simulink model "QuinReader_HW"  (R2023b)
settings: Solver=FixedStepDiscrete  StartTime=0.0  StopTime=5e5*SAMPLE_TIME  RelTol=1e-3
InitFcn:
  | Initialize;
values from neighbouring files (symbols this model uses):
  ALIGN_SIG_LEN = 5000    [Initialize.m]
  BLF = 40e3    (= 40000)    [Initialize.m]
  LPBACK_DECI = designMultirateFIR(1, 2, 0.25, 60,"SystemObject", true)    [Initialize.m]
  NCO = gen_nco_config(SAMPLE_RATE, OperateFreq - CenterFreq)    [Initialize.m]
  SAMPLE_RATE = 122.88e6    (= 122880000)    [Initialize.m]
  SAMPLE_TIME = 1 / SAMPLE_RATE    (= 8.13802083333e-09)    [Initialize.m]
  TX_INTER = designMultirateFIR(2, 1, 0.25, 60,"SystemObject", true)    [Initialize.m]
undefined symbols (not defined in the file or in its folder): ReaderReceive
libraries: hdlsllib x16, simulink x5, dsphdlsigops2 x5, dsphdlfiltering2 x2
CloseFcn:
  | clear rfid rn16 epc rn16_start epc_start
settings Model: DataTypeOverride=Off  Creator=NaXin  LastModifiedBy=NaXin
settings SolverCC: AlgebraicLoopSolver=TrustRegion
settings DataIOCC: LimitDataPoints=on  SaveOutput=off  SaveTime=off
settings OptimizationCC: BlockReduction=off  ConditionallyExecuteInputs=off  DefaultParameterBehavior=Inlined  InheritOutputTypeSmallerThanSingle=on  ReuseModelBlockBuffer=off  LifeSpan=inf
settings DebuggingCC: AlgebraicLoopMsg=error  SingleTaskRateTransMsg=error  UnconnectedInputMsg=warning  UnconnectedOutputMsg=warning  UnconnectedLineMsg=warning  AllowSymbolicDim=off  StrictBusMsg=ErrorOnBusTreatedAsVector  SFUnexpectedBacktrackingDiag=warning  SFNoUnconditionalDefaultTransitionDiag=warning  SFExecutionAtInitializationDiag=none  ArithmeticOperatorsInVariantConditions=warning
settings HardwareCC: ProdBitPerPointer=32  ProdBitPerSizeT=32  ProdBitPerPtrDiffT=32  ProdLargestAtomicFloat=None  ProdIntDivRoundTo=Undefined  ProdEndianess=Unspecified  ProdWordSize=32  ProdHWDeviceType=ASIC/FPGA->ASIC/FPGA  ProdEqTarget=off
settings ModelReferenceCC: EnableRefExpFcnMdlSchedulingChecks=on
settings SFSimCC: SimUseLocalCustomCode=off  CustomCodeUndefinedFunction=UseInterfaceOnly
settings RTWCC: RTWUseLocalCustomCode=off
settings CodeAppCC: StateflowObjectComments=on
settings GRTTargetCC: TargetLangStandard=C89/C90 (ANSI)
settings ConfigComp: CovScope=ReferencedModels  CovMetricSettings=dw  CovSaveCumulativeToWorkspaceVar=on  CovSaveSingleToWorkspaceVar=on  CovExternalEMLEnable=off  CovSFcnEnable=off

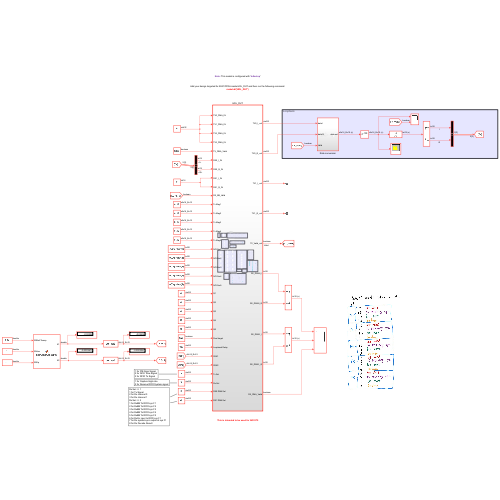
[thumbnail: Simulink's stored preview of the top-level diagram]
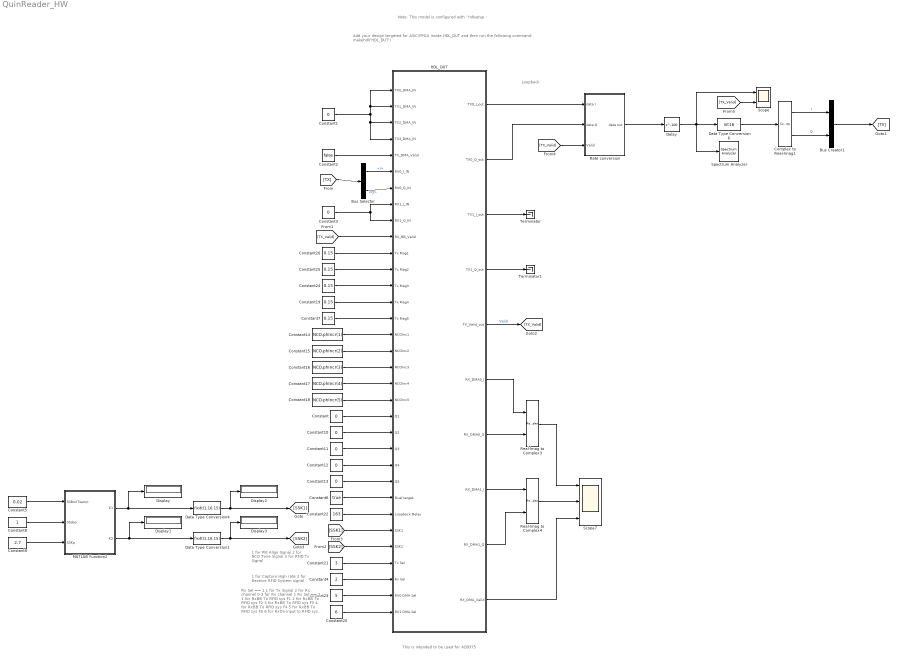
== system QuinReader_HW ==
  note: Note: This model is configured with ' hdlsetup '
  note: Add your design targeted for ASIC/FPGA inside HDL_DUT and then run the following command:
      | makehdl('HDL_DUT')
  note: Rx Sel == 1
      | 1 for Tx Signal
      | 2 for Rx channel 0
      | 3 for Rx channel 1
      | Rx Sel == 2
      | 1 for RxBB To RFID sys F1
      | 2 for RxBB To RFID sys F2
      | 3 for RxBB To RFID sys F3
      | 4 for RxBB To RFID sys F4
      | 5 for RxBB To RFID sys F5
      | 6 for RxOn input to RFID sys F1
      | 7 for Rx symbol sync output at sys F1
      | 8 for Rx Decode Result
  note: 1 for PIE Align Signal
      | 2 for NCO Tone Signal
      | 3 for RFID Tx Signal
  note: Loopback
  note: This is intended to be used for AD9375
  note: 1 for Capture High rate
      | 2 for Receive RFID System signal
  Bus Creator1 : BusCreator  Inputs=2
  Bus Selector : BusSelector  OutputSignals=I,Q
  Complex to Real-Imag1 : ComplexToRealImag
  Constant{,1,10..13} (6 alike) : Constant  Value=0  OutDataTypeStr=uint32  SampleTime=SAMPLE_TIME
  Constant14 : Constant  Value=NCO.phIncr(1)  OutDataTypeStr=int32  SampleTime=SAMPLE_TIME
  Constant15 : Constant  Value=NCO.phIncr(2)  OutDataTypeStr=int32  SampleTime=SAMPLE_TIME
  Constant16 : Constant  Value=NCO.phIncr(3)  OutDataTypeStr=int32  SampleTime=SAMPLE_TIME
  Constant17 : Constant  Value=NCO.phIncr(4)  OutDataTypeStr=int32  SampleTime=SAMPLE_TIME
  Constant18 : Constant  Value=NCO.phIncr(5)  OutDataTypeStr=int32  SampleTime=SAMPLE_TIME
  Constant{7,19,24..26} (5 alike) : Constant  Value=0.15  OutDataTypeStr=fixdt(1,16,15)  SampleTime=SAMPLE_TIME
  Constant2 : Constant  Value=false  OutDataTypeStr=boolean  SampleTime=SAMPLE_TIME
  Constant20 : Constant  Value=6  OutDataTypeStr=uint32  SampleTime=SAMPLE_TIME
  Constant21 : Constant  Value=3  OutDataTypeStr=uint32  SampleTime=SAMPLE_TIME
  Constant22 : Constant  Value=163  OutDataTypeStr=uint32  SampleTime=SAMPLE_TIME
  Constant23 : Constant  Value=5  OutDataTypeStr=uint32  SampleTime=SAMPLE_TIME
  Constant3 : Constant  Value=0  OutDataTypeStr=int16  SampleTime=SAMPLE_TIME
  Constant4 : Constant  Value=2  OutDataTypeStr=uint32  SampleTime=SAMPLE_TIME
  Constant5 : Constant  Value=0.02  SampleTime=SAMPLE_TIME
  Constant6 : Constant  Value=true  OutDataTypeStr=boolean  SampleTime=SAMPLE_TIME
  Constant8 : Constant  SampleTime=SAMPLE_TIME
  Constant9 : Constant  Value=2.7  SampleTime=SAMPLE_TIME
  Data Type Conversion1 : DataTypeConversion  OutDataTypeStr=fixdt(1,16,15)  SaturateOnIntegerOverflow=off  RndMeth=Floor
  Data Type Conversion4 : DataTypeConversion  OutDataTypeStr=fixdt(1,16,15)  SaturateOnIntegerOverflow=off  RndMeth=Floor
  Data Type Conversion6 : DataTypeConversion  OutDataTypeStr=int16  ConvertRealWorld=Stored Integer (SI)  SaturateOnIntegerOverflow=off  RndMeth=Floor
  Delay : Delay  DelayLength=100
  Display{,1..3} (4 alike) : Display
  HDL_DUT : Subsystem  TreatAsAtomicUnit=on
  MATLAB Function2 : MATLAB Function  TreatAsAtomicUnit=on
  Rate conversion : Subsystem
  Real-Imag to Complex3 : RealImagToComplex
  Real-Imag to Complex4 : RealImagToComplex
  Scope : Scope  NumInputPorts=2
  Scope7 : Scope  NumInputPorts=3
  Spectrum Analyzer : SpectrumAnalyzer  WindowPosition=[605.000000,336.000000,800.000000,500.000000,]  ScopeFrameLocation=window  Span=122880000  StartFrequency=-61440000  StopFrequency=61440000  YLimits=[-115.87985262,25.05534256]
      settings: OpenAtSimulationStart=off
  Terminator : Terminator
  Terminator1 : Terminator
  wires:
  Constant2/1 -> HDL_DUT/5(TX_DMA_Valid)
  Constant1/1 -> HDL_DUT/3(TX2_DMA_IN), HDL_DUT/4(TX3_DMA_IN), HDL_DUT/2(TX1_DMA_IN), HDL_DUT/1(TX0_DMA_IN)
  Bus Selector/2 -> HDL_DUT/7(RX0_Q_IN)  "<Q>"
  [TX] -> Bus Selector/1
  Bus Selector/1 -> HDL_DUT/6(RX0_I_IN)  "<I>"
  Constant3/1 -> HDL_DUT/9(RX1_Q_IN), HDL_DUT/8(RX1_I_IN)
  Constant7/1 -> HDL_DUT/15(Tx Mag5)
  Constant/1 -> HDL_DUT/21(Q1)
  Constant20/1 -> HDL_DUT/33(RX1 DMA Sel)
  Constant23/1 -> HDL_DUT/32(RX0 DMA Sel)
  Constant21/1 -> HDL_DUT/30(Tx Sel)
  Constant22/1 -> HDL_DUT/27(Loopback Delay)
  Constant6/1 -> HDL_DUT/26(Dual target)
  Real-Imag to Complex3/1 -> Scope7/1
  HDL_DUT/10(RX_DMA_Valid) -> Scope7/3
  HDL_DUT/9(RX_DMA1_Q) -> Real-Imag to Complex4/2
  Real-Imag to Complex4/1 -> Scope7/2
  HDL_DUT/6(RX_DMA0_I) -> Real-Imag to Complex3/1
  HDL_DUT/8(RX_DMA1_I) -> Real-Imag to Complex4/1
  HDL_DUT/7(RX_DMA0_Q) -> Real-Imag to Complex3/2
  HDL_DUT/3(TX1_I_out) -> Terminator/1
  HDL_DUT/4(TX1_Q_out) -> Terminator1/1
  Bus Creator1/1 -> [TX]
  Complex to Real-Imag1/2 -> Bus Creator1/2  "Q"
  Rate conversion/1(data out) -> Delay/1
  Complex to Real-Imag1/1 -> Bus Creator1/1  "I"
  Data Type Conversion6/1 -> Complex to Real-Imag1/1
  Delay/1 -> Data Type Conversion6/1, Scope/1, Spectrum Analyzer/1
  HDL_DUT/5(TX_Valid_out) -> [TX_Valid]  "Valid"
  [TX_Valid] -> HDL_DUT/10(RX_BB_Valid)
  Constant4/1 -> HDL_DUT/31(Rx Sel)
  Constant5/1 -> MATLAB Function2/1(SSBnXTsamp)
  Constant8/1 -> MATLAB Function2/2(SSdoo)
  Constant9/1 -> MATLAB Function2/3(SSKp)
  MATLAB Function2/2(K2) -> Data Type Conversion1/1, Display1/1
  Data Type Conversion4/1 -> [SSK1], Display2/1
  MATLAB Function2/1(K1) -> Data Type Conversion4/1, Display/1
  Data Type Conversion1/1 -> [SSK2], Display3/1
  [SSK2] -> HDL_DUT/29(SSK2)
  [SSK1] -> HDL_DUT/28(SSK1)
  Constant10/1 -> HDL_DUT/22(Q2)
  Constant11/1 -> HDL_DUT/23(Q3)
  Constant12/1 -> HDL_DUT/24(Q4)
  Constant13/1 -> HDL_DUT/25(Q5)
  Constant14/1 -> HDL_DUT/16(NCOInc1)
  Constant15/1 -> HDL_DUT/17(NCOInc2)
  Constant16/1 -> HDL_DUT/18(NCOInc3)
  Constant17/1 -> HDL_DUT/19(NCOInc4)
  Constant18/1 -> HDL_DUT/20(NCOInc5)
  Constant26/1 -> HDL_DUT/11(Tx Mag1)
  Constant25/1 -> HDL_DUT/12(Tx Mag2)
  Constant24/1 -> HDL_DUT/13(Tx Mag3)
  Constant19/1 -> HDL_DUT/14(Tx Mag4)
  HDL_DUT/1(TX0_I_out) -> Rate conversion/1(data I)
  HDL_DUT/2(TX0_Q_out) -> Rate conversion/2(data Q)
  [TX_Valid] -> Rate conversion/3(Valid)
  [TX_Valid] -> Scope/2

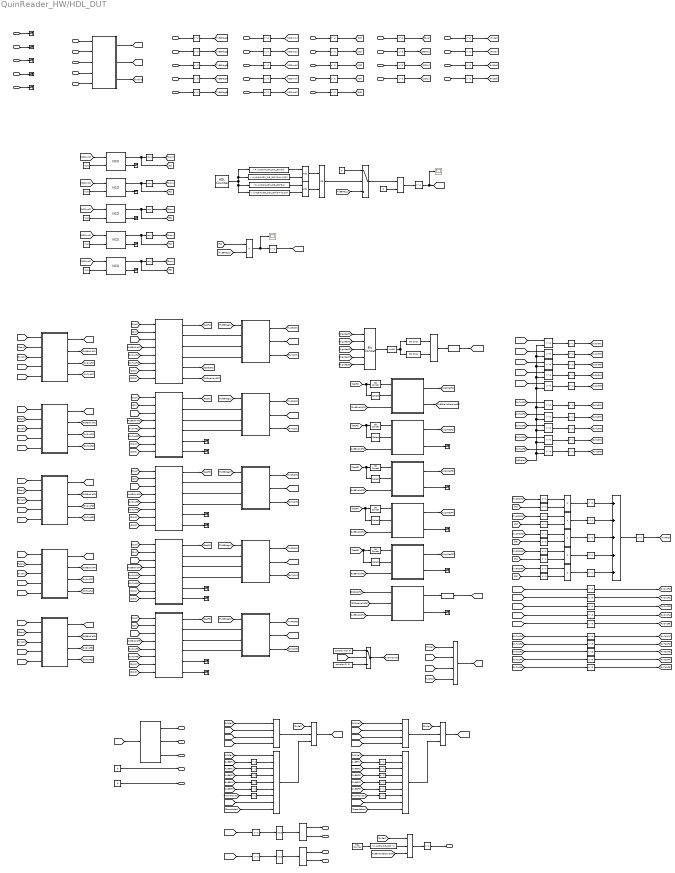
== system QuinReader_HW/HDL_DUT ==
  note: Referenced subsystem RFIDSystem and RFIDRx are exactly the same as in RFID reader. They are actually their copy in QuinReader folder.
  note: Digital up conversion and Tx interpolation
  note: All RxBBValidFx should actually be perfectly aligned.
  note: IF Carrier
  note: Digital down conversion
  note: LoopBack Delay
  note: Unused Tx ports
  note: Input Ports Area
  note: Rx ports and signal prepare
  note: Input Parameters via AXI Lite
  note: Independent Signal Generation
  note: Loopback Delay PIE Signal
  note: Main Signal Tx/Rx Section
  note: Compensate for the loopback delay, including all the way from sending from our IP core to received by our IP core. In other words, the delay includes tx digital sdr part, tx analog part, rf part, rx analog part, rx digital sdr part.
      | Maximum 250 currently, if higher is required, multistage of this must be considered, to maintain the slack time of generated HDL.
  note: Tx Sig Selection
  note: Reader Align Monitor
  note: Output Area
  note: DMA Output
  note: Transmit Signal
  note: Decode result align and merge
  note: RFID system and Tx RC filter
  note: Tone Signal Gen
  TX0_DMA_IN : Inport
  TX1_DMA_IN : Inport  Port=2
  TX2_DMA_IN : Inport  Port=3
  TX3_DMA_IN : Inport  Port=4
  TX_DMA_Valid : Inport  Port=5
  RX0_I_IN : Inport  Port=6
  RX0_Q_IN : Inport  Port=7
  RX1_I_IN : Inport  Port=8
  RX1_Q_IN : Inport  Port=9
  RX_BB_Valid : Inport  Port=10
  Tx Mag1 : Inport  Port=11
  Tx Mag2 : Inport  Port=12
  Tx Mag3 : Inport  Port=13
  Tx Mag4 : Inport  Port=14
  Tx Mag5 : Inport  Port=15
  NCOInc1 : Inport  Port=16
  NCOInc2 : Inport  Port=17
  NCOInc3 : Inport  Port=18
  NCOInc4 : Inport  Port=19
  NCOInc5 : Inport  Port=20
  Q1 : Inport  Port=21
  Q2 : Inport  Port=22
  Q3 : Inport  Port=23
  Q4 : Inport  Port=24
  Q5 : Inport  Port=25
  Dual target : Inport  Port=26
  Loopback Delay : Inport  Port=27
  SSK1 : Inport  Port=28
  SSK2 : Inport  Port=29
  Tx Sel : Inport  Port=30
  Rx Sel : Inport  Port=31
  RX0 DMA Sel : Inport  Port=32
  RX1 DMA Sel : Inport  Port=33
  Add : Sum  Inputs=+++++  OutDataTypeStr=fixdt(1,16,15)  RndMeth=Round  SaturateOnIntegerOverflow=on
  Align Decoded Results F{1..5} (5 alike) : Subsystem  ReferencedSubsystem=Lib_AlignAsyncSignal
  Align SS Out F1 : Subsystem  ReferencedSubsystem=Lib_AlignAsyncSignal
  Bit Concat{1..5} (5 alike) : hdlsllib/Logic and Bit Operations/Bit Concat  numInputs=1
  Bit Concat6 : hdlsllib/Logic and Bit Operations/Bit Concat  numInputs=5
  Bit Slice : hdlsllib/Logic and Bit Operations/Bit Slice  lidx=15  ridx=0
  Bit Slice1 : hdlsllib/Logic and Bit Operations/Bit Slice  lidx=31  ridx=16
  Compare To Constant1 : simulink/Logic and Bit Operations/Compare To Constant  relop=<=  const=ALIGN_SIG_LEN * 2  OutDataTypeStr=boolean
  Compare To Constant2 : simulink/Logic and Bit Operations/Compare To Constant  relop=>=  const=uint16(ALIGN_SIG_LEN*3/4)  OutDataTypeStr=boolean
  Compare To Constant3 : simulink/Logic and Bit Operations/Compare To Constant  relop=<  const=uint16(ALIGN_SIG_LEN*(3/4+1/20))  OutDataTypeStr=boolean
  Compare To Constant4 : simulink/Logic and Bit Operations/Compare To Constant  relop=>=  const=uint16(ALIGN_SIG_LEN*5/4)  OutDataTypeStr=boolean
  Compare To Constant5 : simulink/Logic and Bit Operations/Compare To Constant  relop=<  const=uint16(ALIGN_SIG_LEN*(5/4+1/20))  OutDataTypeStr=boolean
  Complex to Real-Imag3 : ComplexToRealImag
  Complex to Real-Imag4 : ComplexToRealImag
  Constant{,1,3,5..6} (5 alike) : Constant  Value=true  OutDataTypeStr=boolean  SampleTime=SAMPLE_TIME
  Constant13 : Constant  Value=complex(0, 0)  OutDataTypeStr=fixdt(1,16,15)  SampleTime=SAMPLE_TIME
  Constant14 : Constant  Value=complex(0.5, 0)  OutDataTypeStr=fixdt(1,16,15)  SampleTime=SAMPLE_TIME
  Constant2 : Constant  Value=0  OutDataTypeStr=uint32  SampleTime=SAMPLE_TIME
  Constant4 : Constant  Value=0  OutDataTypeStr=uint32  SampleTime=SAMPLE_TIME
  Constant40 : Constant  Value=0  OutDataTypeStr=fixdt(1,16,15)  SampleTime=SAMPLE_TIME
  Constant41 : Constant  Value=0  OutDataTypeStr=fixdt(1,16,15)  SampleTime=SAMPLE_TIME
  DDC F{1..5} (5 alike) : Subsystem  ReferencedSubsystem=Lib_QuinIDRxDDC
  Data Type Conversion : DataTypeConversion  OutDataTypeStr=uint32  SaturateOnIntegerOverflow=off  RndMeth=Floor
  Data Type Conversion1 : DataTypeConversion  OutDataTypeStr=fixdt(1,16,15)  ConvertRealWorld=Stored Integer (SI)  SaturateOnIntegerOverflow=off  RndMeth=Floor
  Data Type Conversion2 : DataTypeConversion  OutDataTypeStr=fixdt(1,16,15)  ConvertRealWorld=Stored Integer (SI)  SaturateOnIntegerOverflow=off  RndMeth=Floor
  Data Type Conversion4 : DataTypeConversion  OutDataTypeStr=int16  ConvertRealWorld=Stored Integer (SI)  SaturateOnIntegerOverflow=off  RndMeth=Floor
  Data Type Conversion5 : DataTypeConversion  OutDataTypeStr=int16  ConvertRealWorld=Stored Integer (SI)  SaturateOnIntegerOverflow=off  RndMeth=Floor
  Delay{,3..12,18,20..30} (23 alike) : Delay
  Delay{1,40,42,44,46} (5 alike) : Delay  DelayLengthSource=Input port  DelayLengthUpperLimit=250  InitialCondition=ReaderReceive.RN16  DiagnosticForDelayLength=Error  UseCircularBuffer=on
      settings: InputPortMap=u0,p1
  Delay{13..14,19,48..63,73..84,93} (32 alike) : Delay  DelayLength=1
  Delay{15..16,32,34,36,38} (6 alike) : Delay  DelayLength=1  InitialCondition=false
  Delay{17,41,43,45,47} (5 alike) : Delay  DelayLength=1  InitialCondition=ReaderReceive.RN16
  Delay{2,33,35,37,39} (5 alike) : Delay  DelayLengthSource=Input port  DelayLengthUpperLimit=250  InitialCondition=false  DiagnosticForDelayLength=Error  UseCircularBuffer=on
      settings: InputPortMap=u0,p1
  Delay{31,64..67} (5 alike) : Delay  DelayLength=3  InitialCondition=false
  Delay{68..72} (5 alike) : Delay  DelayLength=3  InitialCondition=ReaderReceive.RN16
  HDL Counter2 : hdlsllib/Sources/HDL Counter  CountType=Count limited  CountInit=1  CountStep=1  CountMax=2*ALIGN_SIG_LEN  CountFromType=Initial value  CountFrom=1  CountResetPort=off  CountLoadPort=off  CountEnbPort=off  CountDirPort=off  CountHitOutputPort=off  CountDataType=Unsigned  CountWordLen=16  CountFracLen=0  CountSampTime=SAMPLE_TIME
  HDL Counter4 : hdlsllib/Sources/HDL Counter  CountType=Count limited  CountInit=1  CountStep=1  CountMax=SAMPLE_RATE / (8 * BLF) * ALIGN_SIG_LEN * 2  CountFromType=Initial value  CountFrom=1  CountResetPort=off  CountLoadPort=off  CountEnbPort=off  CountDirPort=off  CountHitOutputPort=off  CountDataType=Unsigned  CountWordLen=32  CountFracLen=0  CountSampTime=SAMPLE_TIME
  Logical Operator10 : Logic  AllPortsSameDT=off  OutDataTypeStr=boolean
  Logical Operator11 : Logic  AllPortsSameDT=off  OutDataTypeStr=boolean
  Logical Operator12 : Logic  Operator=OR  AllPortsSameDT=off  OutDataTypeStr=boolean
  Math Function{,1..4} (5 alike) : Math  Operator=conj  SignedPower=on  RndMeth=Zero  SaturateOnIntegerOverflow=off
  Multiport Switch1 : MultiPortSwitch  Inputs=2  DataPortIndices={[1,2,3,4],5}  DiagnosticForDefault=None  SaturateOnIntegerOverflow=off  InputSameDT=off
  Multiport Switch2 : MultiPortSwitch  Inputs=2  DataPortIndices={[1,2,3,4],5}  DiagnosticForDefault=None  SaturateOnIntegerOverflow=off  InputSameDT=off
  Multiport Switch3 : MultiPortSwitch  Inputs=8  DataPortIndices={[1,2,3,4],5}  DiagnosticForDefault=None  SaturateOnIntegerOverflow=off  InputSameDT=off
  Multiport Switch4 : MultiPortSwitch  DiagnosticForDefault=None  SaturateOnIntegerOverflow=off  InputSameDT=off
  Multiport Switch5 : MultiPortSwitch  Inputs=8  DataPortIndices={[1,2,3,4],5}  DiagnosticForDefault=None  SaturateOnIntegerOverflow=off  InputSameDT=off
  Multiport Switch6 : MultiPortSwitch  DataPortIndices={[1,2,3,4],5}  DiagnosticForDefault=None  SaturateOnIntegerOverflow=off  InputSameDT=off
  Multiport Switch7 : MultiPortSwitch  DataPortIndices={[1,2,3,4],5}  DiagnosticForDefault=None  SaturateOnIntegerOverflow=off  InputSameDT=off
  Multiport Switch8 : MultiPortSwitch  Inputs=2  DataPortIndices={[1,2,3,4],5}  DiagnosticForDefault=None  SaturateOnIntegerOverflow=off  InputSameDT=off
  NCO F{1..5} (5 alike) : dsphdlsigops2/NCO  PhaseIncrementSource=Input port  PhaseIncrement=100  PhaseOffsetSource=Property  PhaseOffset=0  DitherSource=Property  NumDitherBits=NCO.ditherBits  SamplesPerFrame=1  LUTCompress=off  ResetAction=off  Waveform=Complex exponential  PhasePort=off  SimulateUsing=Code generation  AccumulatorWL=NCO.N  PhaseQuantization=on  NumQuantizerAccumulatorBits=NCO.Q  OutputDataType=Binary point scaling  OutputWL=16  OutputFL=14
      settings: LibrarySourceBlock=dsphdlsrcs2/NCO
  Prepare Input : Subsystem
  Product{,1..2,4..5} (5 alike) : Product  RndMeth=Round  OutDataTypeStr=Inherit: Same as first input
  Product3 : Product  OutDataTypeStr=fixdt(1,16,15)  RndMeth=Round
  RFID System F{1..5} (5 alike) : Subsystem  ReferencedSubsystem=Lib_RFIDSystem
  Real-Imag to Complex2 : RealImagToComplex
  Real-Imag to Complex6 : RealImagToComplex
  Scope4 : Scope  Commented=on
  Scope5 : Scope  Commented=on
  Selector{1..5} (5 alike) : Selector  InputPortWidth=4  IndexOptions=Index vector (dialog)  Indices=[1]  OutputSizes=1
  Switch5 : Switch  Criteria=u2 > Threshold  SaturateOnIntegerOverflow=off  InputSameDT=off
  Switch6 : Switch  Criteria=u2 > Threshold  SaturateOnIntegerOverflow=off  InputSameDT=off
  TX Prepare : Subsystem
  Terminator{,1..22} (23 alike) : Terminator
  Tx Filter F{1..5} (5 alike) : Subsystem  ReferencedSubsystem=Lib_QuinIDTxFilter
  TX0_I_out : Outport
  TX0_Q_out : Outport  Port=2
  TX1_I_out : Outport  Port=3
  TX1_Q_out : Outport  Port=4
  TX_Valid_out : Outport  Port=5
  RX_DMA0_I : Outport  Port=6
  RX_DMA0_Q : Outport  Port=7
  RX_DMA1_I : Outport  Port=8
  RX_DMA1_Q : Outport  Port=9
  RX_DMA_Valid : Outport  Port=10
  wires:
  TX2_DMA_IN/1 -> Terminator12/1
  TX3_DMA_IN/1 -> Terminator13/1
  TX_DMA_Valid/1 -> Terminator11/1
  TX1_DMA_IN/1 -> Terminator10/1
  TX0_DMA_IN/1 -> Terminator9/1
  Prepare Input/1(data0 out) -> [RxData0]
  Prepare Input/3(valid out) -> [RxValid]
  Prepare Input/2(data1 out) -> [RxData1]
  RX1_I_IN/1 -> Prepare Input/3(data I1)
  RX0_I_IN/1 -> Prepare Input/1(data I0)
  RX1_Q_IN/1 -> Prepare Input/4(data Q1)
  RX0_Q_IN/1 -> Prepare Input/2(data Q0)
  RX_BB_Valid/1 -> Prepare Input/5(data valid)
  Tx Mag1/1 -> Delay/1
  Q1/1 -> Delay3/1
  Tx Sel/1 -> Delay6/1
  Loopback Delay/1 -> Delay5/1
  RX0 DMA Sel/1 -> Delay8/1
  RX1 DMA Sel/1 -> Delay9/1
  Dual target/1 -> Delay4/1
  Real-Imag to Complex2/1 -> Delay19/1
  Compare To Constant3/1 -> Logical Operator10/2
  [TxBBMag1] -> Switch5/3
  HDL Counter2/1 -> Compare To Constant3/1, Compare To Constant2/1, Compare To Constant4/1, Compare To Constant5/1
  Constant40/1 -> Switch5/1
  Logical Operator12/1 -> Switch5/2
  Compare To Constant4/1 -> Logical Operator11/1
  Logical Operator11/1 -> Logical Operator12/2
  Switch5/1 -> Real-Imag to Complex2/1
  Constant41/1 -> Real-Imag to Complex2/2
  Compare To Constant2/1 -> Logical Operator10/1
  Compare To Constant5/1 -> Logical Operator11/2
  Logical Operator10/1 -> Logical Operator12/1
  [Dual] -> RFID System F1/1
  [Q1] -> RFID System F1/2
  RFID System F1/1 -> [ResF1]
  [RxOn2F1] -> Delay2/1
  [RxTp2F1] -> Delay1/1
  [RxOn4F1] -> RFID System F1/5
  [RxTp4F1] -> RFID System F1/6
  Delay2/1 -> Delay16/1
  Delay1/1 -> Delay17/1
  [LBDelay] -> Delay46/2, Delay44/2, Delay40/2, Delay1/2, Delay39/2, Delay37/2, Delay35/2, Delay33/2, Delay2/2, Delay42/2
  Constant14/1 -> Switch6/1
  Constant13/1 -> Switch6/3
  [RxOn4F1] -> Switch6/2
  Switch6/1 -> [RxOnMonitor]
  [AlignSig] -> Multiport Switch4/2
  [TxSel] -> Multiport Switch4/1
  [TxRFID] -> Multiport Switch4/4
  Multiport Switch4/1 -> [TxData]  "data_in"
  Data Type Conversion5/1 -> Complex to Real-Imag4/1
  Complex to Real-Imag3/2 -> RX_DMA0_Q/1
  Multiport Switch6/1 -> Multiport Switch2/2
  Constant2/1 -> TX1_I_out/1
  TX Prepare/3(data valid) -> TX_Valid_out/1
  Complex to Real-Imag4/1 -> RX_DMA1_I/1
  [DMAOut0] -> Delay13/1
  [DecodeRes] -> Multiport Switch5/9
  Complex to Real-Imag3/1 -> RX_DMA0_I/1
  TX Prepare/1(data I out) -> TX0_I_out/1
  Constant4/1 -> TX1_Q_out/1
  Data Type Conversion4/1 -> Complex to Real-Imag3/1
  TX Prepare/2(data Q out) -> TX0_Q_out/1
  [RxOnMonitor] -> Delay84/1
  [DMAOut1] -> Delay14/1
  Complex to Real-Imag4/2 -> RX_DMA1_Q/1
  [RxBBF1] -> Delay79/1
  Bit Slice/1 -> Real-Imag to Complex6/2
  Data Type Conversion/1 -> Bit Slice/1, Bit Slice1/1
  Bit Slice1/1 -> Real-Imag to Complex6/1
  Real-Imag to Complex6/1 -> Data Type Conversion2/1
  Data Type Conversion2/1 -> [DecodeRes]
  [TxBBMag1] -> Tx Filter F1/1
  RFID System F1/2 -> Tx Filter F1/2
  RFID System F1/3 -> Tx Filter F1/3
  RFID System F1/4 -> Tx Filter F1/4
  Tx Filter F1/1 -> [TxRFIDF1]
  Tx Filter F1/2 -> [RxOn1F1]
  Tx Filter F1/3 -> [RxTp1F1]
  [RxData0] -> DDC F1/1
  [RxValid] -> DDC F1/3
  [RxTp3F1] -> DDC F1/5
  [RxOn3F1] -> DDC F1/4
  DDC F1/1 -> [RxBBF1]
  DDC F1/2 -> [RxBBValidF1]
  DDC F1/4 -> [RxTp4F1]
  DDC F1/3 -> [RxOn4F1]
  [RxBBF1] -> RFID System F1/3
  [RxBBValidF1] -> RFID System F1/4
  [RxData1] -> Multiport Switch6/4
  [RxData0] -> Multiport Switch6/3
  [RX0Sel] -> Multiport Switch6/1
  [TxData] -> Multiport Switch6/2
  HDL Counter4/1 -> Compare To Constant1/1
  Rx Sel/1 -> Delay7/1
  [RX0Sel] -> Multiport Switch5/1
  [RxSel] -> Multiport Switch2/1
  Multiport Switch5/1 -> Multiport Switch2/3
  Multiport Switch2/1 -> [DMAOut0]
  Multiport Switch7/1 -> Multiport Switch1/2
  [RX1Sel] -> Multiport Switch3/1
  [RxData1] -> Multiport Switch7/4
  Multiport Switch3/1 -> Multiport Switch1/3
  [DecodeRes] -> Multiport Switch3/9
  [RX1Sel] -> Multiport Switch7/1
  [RxBBF1] -> Delay73/1
  Multiport Switch1/1 -> [DMAOut1]
  [RxData0] -> Multiport Switch7/3
  [TxData] -> Multiport Switch7/2
  [RxSel] -> Multiport Switch1/1
  [RxOnMonitor] -> Delay78/1
  Compare To Constant1/1 -> Multiport Switch8/2
  Multiport Switch8/1 -> Delay15/1
  [RxSel] -> Multiport Switch8/1
  [RxBBValidF1] -> Align Decoded Results F1/3
  Bit Concat6/1 -> Data Type Conversion/1
  Delay/1 -> [TxBBMag1]
  Delay3/1 -> [Q1]
  Delay4/1 -> [Dual]
  Delay6/1 -> [TxSel]
  Delay7/1 -> [RxSel]
  Delay8/1 -> [RX0Sel]
  Delay9/1 -> [RX1Sel]
  SSK1/1 -> Delay10/1
  Delay10/1 -> [SSK1]
  SSK2/1 -> Delay11/1
  Delay11/1 -> [SSK2]
  RFID System F1/6 -> [SSDataValidF1]
  RFID System F1/5 -> [SSDataF1]
  [SSK1] -> RFID System F1/7
  [SSK2] -> RFID System F1/8
  [SSDataF1] -> Align SS Out F1/1
  [SSDataValidF1] -> Align SS Out F1/2
  [RxBBValidF1] -> Align SS Out F1/3
  Align SS Out F1/1 -> Data Type Conversion1/1
  Data Type Conversion1/1 -> [SSOutput]
  [SSOutput] -> Multiport Switch5/8
  [SSOutput] -> Multiport Switch3/8
  Delay13/1 -> Data Type Conversion4/1
  Delay14/1 -> Data Type Conversion5/1
  Delay15/1 -> RX_DMA_Valid/1
  Delay16/1 -> [RxOn3F1]
  Delay17/1 -> [RxTp3F1]
  Delay19/1 -> [AlignSig], Scope5/1
  Delay5/1 -> [LBDelay]
  Tx Mag2/1 -> Delay12/1
  Delay12/1 -> [TxBBMag2]
  Tx Mag3/1 -> Delay18/1
  Delay18/1 -> [TxBBMag3]
  Tx Mag4/1 -> Delay20/1
  Delay20/1 -> [TxBBMag4]
  Tx Mag5/1 -> Delay21/1
  Delay21/1 -> [TxBBMag5]
  Delay25/1 -> [NCOInc4]
  NCOInc4/1 -> Delay25/1
  NCOInc1/1 -> Delay22/1
  Delay22/1 -> [NCOInc1]
  Delay26/1 -> [NCOInc5]
  Delay24/1 -> [NCOInc3]
  Delay23/1 -> [NCOInc2]
  NCOInc5/1 -> Delay26/1
  NCOInc3/1 -> Delay24/1
  NCOInc2/1 -> Delay23/1
  Delay27/1 -> [Q2]
  Q2/1 -> Delay27/1
  Delay28/1 -> [Q3]
  Q3/1 -> Delay28/1
  Delay29/1 -> [Q4]
  Q4/1 -> Delay29/1
  Delay30/1 -> [Q5]
  Q5/1 -> Delay30/1
  Constant/1 -> NCO F1/2
  [NCOInc1] -> NCO F1/1
  NCO F1/2 -> Terminator/1
  NCO F1/1 -> [F1], Math Function/1
  Math Function/1 -> [F1conj]
  [NCOInc2] -> NCO F2/1
  NCO F2/1 -> [F2], Math Function1/1
  Constant1/1 -> NCO F2/2
  NCO F2/2 -> Terminator1/1
  Math Function1/1 -> [F2conj]
  [NCOInc3] -> NCO F3/1
  NCO F3/1 -> [F3], Math Function2/1
  Constant3/1 -> NCO F3/2
  NCO F3/2 -> Terminator2/1
  Math Function2/1 -> [F3conj]
  [NCOInc4] -> NCO F4/1
  NCO F4/1 -> [F4], Math Function3/1
  Constant5/1 -> NCO F4/2
  NCO F4/2 -> Terminator3/1
  Math Function3/1 -> [F4conj]
  [NCOInc5] -> NCO F5/1
  NCO F5/1 -> [F5], Math Function4/1
  Constant6/1 -> NCO F5/2
  NCO F5/2 -> Terminator4/1
  Math Function4/1 -> [F5conj]
  [F1conj] -> DDC F1/2
  DDC F2/1 -> [RxBBF2]
  DDC F2/2 -> [RxBBValidF2]
  [RxValid] -> DDC F2/3
  DDC F2/3 -> [RxOn4F2]
  [RxOn3F2] -> DDC F2/4
  [RxTp3F2] -> DDC F2/5
  [RxData0] -> DDC F2/1
  [F2conj] -> DDC F2/2
  DDC F2/4 -> [RxTp4F2]
  DDC F3/1 -> [RxBBF3]
  DDC F3/2 -> [RxBBValidF3]
  [RxValid] -> DDC F3/3
  DDC F3/3 -> [RxOn4F3]
  [RxOn3F3] -> DDC F3/4
  [RxTp3F3] -> DDC F3/5
  [RxData0] -> DDC F3/1
  [F3conj] -> DDC F3/2
  DDC F3/4 -> [RxTp4F3]
  DDC F4/1 -> [RxBBF4]
  DDC F4/2 -> [RxBBValidF4]
  [RxValid] -> DDC F4/3
  DDC F4/3 -> [RxOn4F4]
  [RxOn3F4] -> DDC F4/4
  [RxTp3F4] -> DDC F4/5
  [RxData0] -> DDC F4/1
  [F4conj] -> DDC F4/2
  DDC F4/4 -> [RxTp4F4]
  DDC F5/1 -> [RxBBF5]
  DDC F5/2 -> [RxBBValidF5]
  [RxValid] -> DDC F5/3
  DDC F5/3 -> [RxOn4F5]
  [RxOn3F5] -> DDC F5/4
  [RxTp3F5] -> DDC F5/5
  [RxData0] -> DDC F5/1
  [F5conj] -> DDC F5/2
  DDC F5/4 -> [RxTp4F5]
  [RxBBF2] -> RFID System F2/3
  [RxBBValidF2] -> RFID System F2/4
  [TxBBMag2] -> Tx Filter F2/1
  RFID System F2/2 -> Tx Filter F2/2
  RFID System F2/5 -> Terminator7/1
  RFID System F2/6 -> Terminator8/1
  [Q2] -> RFID System F2/2
  [RxOn4F2] -> RFID System F2/5
  Tx Filter F2/3 -> [RxTp1F2]
  RFID System F2/4 -> Tx Filter F2/4
  [RxTp4F2] -> RFID System F2/6
  [SSK2] -> RFID System F2/8
  Tx Filter F2/2 -> [RxOn1F2]
  RFID System F2/3 -> Tx Filter F2/3
  [SSK1] -> RFID System F2/7
  Tx Filter F2/1 -> [TxRFIDF2]
  RFID System F2/1 -> [ResF2]
  [Dual] -> RFID System F2/1
  [RxBBF3] -> RFID System F3/3
  [RxBBValidF3] -> RFID System F3/4
  [TxBBMag3] -> Tx Filter F3/1
  RFID System F3/2 -> Tx Filter F3/2
  RFID System F3/5 -> Terminator14/1
  RFID System F3/6 -> Terminator15/1
  [Q3] -> RFID System F3/2
  [RxOn4F3] -> RFID System F3/5
  Tx Filter F3/3 -> [RxTp1F3]
  RFID System F3/4 -> Tx Filter F3/4
  [RxTp4F3] -> RFID System F3/6
  [SSK2] -> RFID System F3/8
  Tx Filter F3/2 -> [RxOn1F3]
  RFID System F3/3 -> Tx Filter F3/3
  [SSK1] -> RFID System F3/7
  Tx Filter F3/1 -> [TxRFIDF3]
  RFID System F3/1 -> [ResF3]
  [Dual] -> RFID System F3/1
  [RxBBF4] -> RFID System F4/3
  [RxBBValidF4] -> RFID System F4/4
  [TxBBMag4] -> Tx Filter F4/1
  RFID System F4/2 -> Tx Filter F4/2
  RFID System F4/5 -> Terminator16/1
  RFID System F4/6 -> Terminator17/1
  [Q4] -> RFID System F4/2
  [RxOn4F4] -> RFID System F4/5
  Tx Filter F4/3 -> [RxTp1F4]
  RFID System F4/4 -> Tx Filter F4/4
  [RxTp4F4] -> RFID System F4/6
  [SSK2] -> RFID System F4/8
  Tx Filter F4/2 -> [RxOn1F4]
  RFID System F4/3 -> Tx Filter F4/3
  [SSK1] -> RFID System F4/7
  Tx Filter F4/1 -> [TxRFIDF4]
  RFID System F4/1 -> [ResF4]
  [Dual] -> RFID System F4/1
  [RxBBF5] -> RFID System F5/3
  [RxBBValidF5] -> RFID System F5/4
  [TxBBMag5] -> Tx Filter F5/1
  RFID System F5/2 -> Tx Filter F5/2
  RFID System F5/5 -> Terminator18/1
  RFID System F5/6 -> Terminator19/1
  [Q5] -> RFID System F5/2
  [RxOn4F5] -> RFID System F5/5
  Tx Filter F5/3 -> [RxTp1F5]
  RFID System F5/4 -> Tx Filter F5/4
  [RxTp4F5] -> RFID System F5/6
  [SSK2] -> RFID System F5/8
  Tx Filter F5/2 -> [RxOn1F5]
  RFID System F5/3 -> Tx Filter F5/3
  [SSK1] -> RFID System F5/7
  Tx Filter F5/1 -> [TxRFIDF5]
  RFID System F5/1 -> [ResF5]
  [Dual] -> RFID System F5/1
  Delay32/1 -> [RxOn3F2]
  Delay33/1 -> Delay32/1
  [RxOn2F2] -> Delay33/1
  Delay35/1 -> Delay34/1
  [RxOn2F3] -> Delay35/1
  Delay34/1 -> [RxOn3F3]
  Delay37/1 -> Delay36/1
  [RxOn2F4] -> Delay37/1
  Delay36/1 -> [RxOn3F4]
  Delay39/1 -> Delay38/1
  [RxOn2F5] -> Delay39/1
  Delay38/1 -> [RxOn3F5]
  Delay41/1 -> [RxTp3F2]
  [RxTp2F2] -> Delay40/1
  Delay40/1 -> Delay41/1
  Delay43/1 -> [RxTp3F3]
  [RxTp2F3] -> Delay42/1
  Delay42/1 -> Delay43/1
  Delay45/1 -> [RxTp3F4]
  [RxTp2F4] -> Delay44/1
  Delay44/1 -> Delay45/1
  Delay47/1 -> [RxTp3F5]
  [RxTp2F5] -> Delay46/1
  Delay46/1 -> Delay47/1
  [F1] -> Delay49/1
  [TxRFIDF1] -> Delay48/1
  [TxRFIDF2] -> Delay50/1
  [TxRFIDF3] -> Delay52/1
  [TxRFIDF4] -> Delay54/1
  [TxRFIDF5] -> Delay56/1
  [F2] -> Delay51/1
  [F3] -> Delay53/1
  [F4] -> Delay55/1
  [F5] -> Delay57/1
  Delay48/1 -> Product/1
  Delay49/1 -> Product/2
  Delay50/1 -> Product1/1
  Delay51/1 -> Product1/2
  Delay52/1 -> Product2/1
  Delay53/1 -> Product2/2
  Delay54/1 -> Product4/1
  Delay55/1 -> Product4/2
  Delay56/1 -> Product5/1
  Delay57/1 -> Product5/2
  Product/1 -> Delay58/1
  Product1/1 -> Delay59/1
  Product2/1 -> Delay60/1
  Product4/1 -> Delay61/1
  Product5/1 -> Delay62/1
  Delay59/1 -> Add/2
  Delay58/1 -> Add/1
  Delay60/1 -> Add/3
  Delay61/1 -> Add/4
  Delay62/1 -> Add/5
  Add/1 -> Delay63/1
  Delay63/1 -> [TxRFID]
  [RxOn1F1] -> Delay31/1
  [RxOn1F2] -> Delay64/1
  [RxOn1F3] -> Delay65/1
  [RxOn1F4] -> Delay66/1
  [RxOn1F5] -> Delay67/1
  [RxTp1F1] -> Delay68/1
  [RxTp1F2] -> Delay69/1
  [RxTp1F3] -> Delay70/1
  [RxTp1F4] -> Delay71/1
  [RxTp1F5] -> Delay72/1
  Delay31/1 -> [RxOn2F1]
  Delay64/1 -> [RxOn2F2]
  Delay65/1 -> [RxOn2F3]
  Delay66/1 -> [RxOn2F4]
  Delay67/1 -> [RxOn2F5]
  Delay68/1 -> [RxTp2F1]
  Delay69/1 -> [RxTp2F2]
  Delay70/1 -> [RxTp2F3]
  Delay71/1 -> [RxTp2F4]
  Delay72/1 -> [RxTp2F5]
  [ResF1] -> Selector1/1, Bit Concat1/1
  [ResF2] -> Selector2/1, Bit Concat2/1
  [ResF3] -> Selector3/1, Bit Concat3/1
  [ResF5] -> Selector5/1, Bit Concat5/1
  [ResF4] -> Selector4/1, Bit Concat4/1
  [RxBBF5] -> Delay83/1
  [RxBBF4] -> Delay82/1
  [RxBBF3] -> Delay81/1
  [RxBBF2] -> Delay80/1
  [RxBBF5] -> Delay77/1
  [RxBBF4] -> Delay76/1
  [RxBBF3] -> Delay75/1
  [RxBBF2] -> Delay74/1
  [TxData] -> TX Prepare/1(data in)
  Product3/1 -> Scope4/1, Delay93/1
  [TxBBMag1] -> Product3/2
  Delay93/1 -> [ToneSig]
  [F1] -> Product3/1
  [ToneSig] -> Multiport Switch4/3
  Bit Concat1/1 -> Align Decoded Results F1/1
  Selector1/1 -> Align Decoded Results F1/2
  Align Decoded Results F1/2 -> [RxBBValidDelayedF1]
  Bit Concat2/1 -> Align Decoded Results F2/1
  Selector2/1 -> Align Decoded Results F2/2
  Bit Concat3/1 -> Align Decoded Results F3/1
  Selector3/1 -> Align Decoded Results F3/2
  Bit Concat4/1 -> Align Decoded Results F4/1
  Selector4/1 -> Align Decoded Results F4/2
  Bit Concat5/1 -> Align Decoded Results F5/1
  Selector5/1 -> Align Decoded Results F5/2
  [RxBBValidF2] -> Align Decoded Results F2/3
  [RxBBValidF3] -> Align Decoded Results F3/3
  [RxBBValidF4] -> Align Decoded Results F4/3
  [RxBBValidF5] -> Align Decoded Results F5/3
  Align Decoded Results F2/2 -> Terminator5/1
  Align Decoded Results F3/2 -> Terminator6/1
  Align Decoded Results F4/2 -> Terminator20/1
  Align Decoded Results F5/2 -> Terminator21/1
  Align Decoded Results F1/1 -> [AlignResF1]
  Align Decoded Results F2/1 -> [AlignResF2]
  Align Decoded Results F3/1 -> [AlignResF3]
  Align Decoded Results F4/1 -> [AlignResF4]
  Align Decoded Results F5/1 -> [AlignResF5]
  [AlignResF1] -> Bit Concat6/1
  [AlignResF2] -> Bit Concat6/2
  [AlignResF3] -> Bit Concat6/3
  [AlignResF4] -> Bit Concat6/4
  [AlignResF5] -> Bit Concat6/5
  Align SS Out F1/2 -> Terminator22/1
  [RxBBValidDelayedF1] -> Multiport Switch8/3
  Delay73/1 -> Multiport Switch3/2
  Delay74/1 -> Multiport Switch3/3
  Delay75/1 -> Multiport Switch3/4
  Delay76/1 -> Multiport Switch3/5
  Delay77/1 -> Multiport Switch3/6
  Delay78/1 -> Multiport Switch3/7
  Delay79/1 -> Multiport Switch5/2
  Delay80/1 -> Multiport Switch5/3
  Delay81/1 -> Multiport Switch5/4
  Delay82/1 -> Multiport Switch5/5
  Delay83/1 -> Multiport Switch5/6
  Delay84/1 -> Multiport Switch5/7

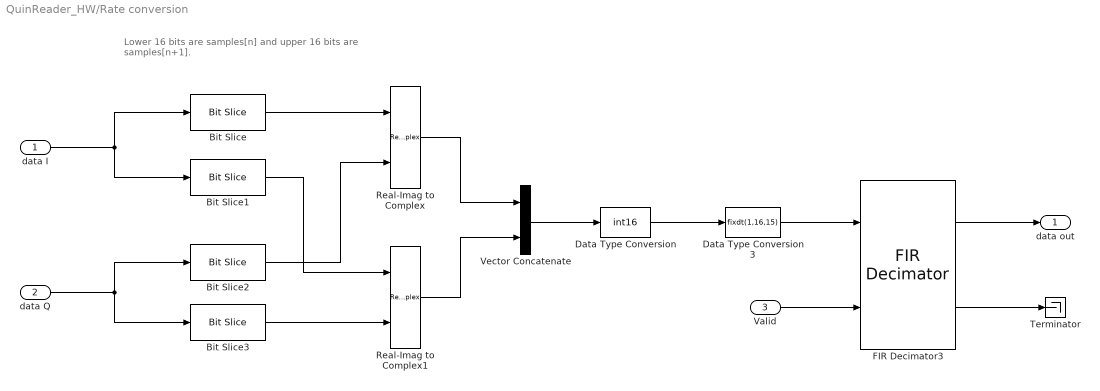
== system QuinReader_HW/Rate conversion ==
  note: Lower 16 bits are samples[n] and upper 16 bits are samples[n+1].
  data I : Inport
  data Q : Inport  Port=2
  Valid : Inport  Port=3
  Bit Slice : hdlsllib/Logic and Bit Operations/Bit Slice  lidx=15  ridx=0
  Bit Slice1 : hdlsllib/Logic and Bit Operations/Bit Slice  lidx=31  ridx=16
  Bit Slice2 : hdlsllib/Logic and Bit Operations/Bit Slice  lidx=15  ridx=0
  Bit Slice3 : hdlsllib/Logic and Bit Operations/Bit Slice  lidx=31  ridx=16
  Data Type Conversion : DataTypeConversion  OutDataTypeStr=int16  ConvertRealWorld=Stored Integer (SI)  SaturateOnIntegerOverflow=off  RndMeth=Floor
  Data Type Conversion3 : DataTypeConversion  OutDataTypeStr=fixdt(1,16,15)  ConvertRealWorld=Stored Integer (SI)  SaturateOnIntegerOverflow=off  RndMeth=Floor
  FIR Decimator3 : dsphdlfiltering2/FIR Decimator  Numerator=LPBACK_DECI.Numerator  FilterStructure=Direct form systolic  DecimationFactor=LPBACK_DECI.DecimationFactor  NumCycles=1  SimulateUsing=Code generation  roundingMode=Round  overflowMode=on  CoefficientsDataTypeStr=fixdt(1,16,15)  OutputDataTypeStr=fixdt(1,16,15)  ResetInputPort=off  HDLGlobalReset=off
  Real-Imag to Complex : RealImagToComplex
  Real-Imag to Complex1 : RealImagToComplex
  Terminator : Terminator
  Vector Concatenate : Concatenate
  data out : Outport
  wires:
  Real-Imag to Complex/1 -> Vector Concatenate/1
  Bit Slice2/1 -> Real-Imag to Complex/2
  Bit Slice/1 -> Real-Imag to Complex/1
  data Q/1 -> Bit Slice3/1, Bit Slice2/1
  data I/1 -> Bit Slice1/1, Bit Slice/1
  Bit Slice3/1 -> Real-Imag to Complex1/2
  Bit Slice1/1 -> Real-Imag to Complex1/1
  Real-Imag to Complex1/1 -> Vector Concatenate/2
  Vector Concatenate/1 -> Data Type Conversion/1
  Valid/1 -> FIR Decimator3/2
  FIR Decimator3/2 -> Terminator/1
  FIR Decimator3/1 -> data out/1
  Data Type Conversion/1 -> Data Type Conversion3/1
  Data Type Conversion3/1 -> FIR Decimator3/1

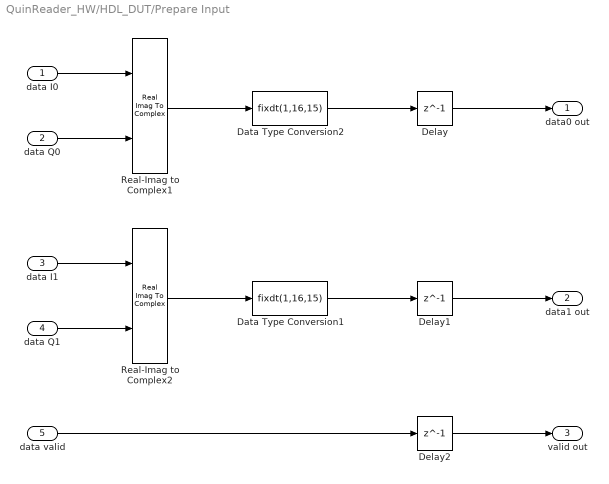
== system QuinReader_HW/HDL_DUT/Prepare Input ==
  data I0 : Inport
  data Q0 : Inport  Port=2
  data I1 : Inport  Port=3
  data Q1 : Inport  Port=4
  data valid : Inport  Port=5
  Data Type Conversion1 : DataTypeConversion  OutDataTypeStr=fixdt(1,16,15)  ConvertRealWorld=Stored Integer (SI)  SaturateOnIntegerOverflow=off  RndMeth=Floor
  Data Type Conversion2 : DataTypeConversion  OutDataTypeStr=fixdt(1,16,15)  ConvertRealWorld=Stored Integer (SI)  SaturateOnIntegerOverflow=off  RndMeth=Floor
  Delay : Delay  DelayLength=1
  Delay1 : Delay  DelayLength=1
  Delay2 : Delay  DelayLength=1  InitialCondition=false
  Real-Imag to Complex1 : RealImagToComplex
  Real-Imag to Complex2 : RealImagToComplex
  data0 out : Outport
  data1 out : Outport  Port=2
  valid out : Outport  Port=3
  wires:
  data Q1/1 -> Real-Imag to Complex2/2
  Real-Imag to Complex1/1 -> Data Type Conversion2/1
  data I0/1 -> Real-Imag to Complex1/1
  data Q0/1 -> Real-Imag to Complex1/2
  Real-Imag to Complex2/1 -> Data Type Conversion1/1
  data I1/1 -> Real-Imag to Complex2/1
  data valid/1 -> Delay2/1
  Data Type Conversion2/1 -> Delay/1
  Data Type Conversion1/1 -> Delay1/1
  Delay/1 -> data0 out/1
  Delay1/1 -> data1 out/1
  Delay2/1 -> valid out/1

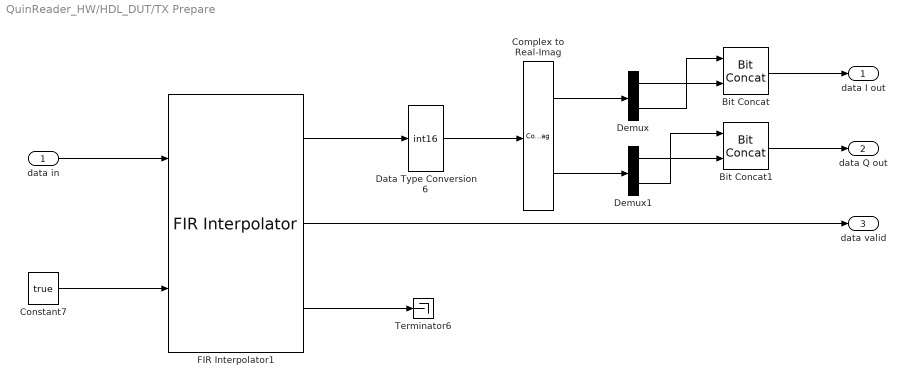
== system QuinReader_HW/HDL_DUT/TX Prepare ==
  data in : Inport
  Bit Concat : hdlsllib/Logic and Bit Operations/Bit Concat  numInputs=2
  Bit Concat1 : hdlsllib/Logic and Bit Operations/Bit Concat  numInputs=2
  Complex to Real-Imag : ComplexToRealImag
  Constant7 : Constant  Value=true  OutDataTypeStr=boolean  SampleTime=SAMPLE_TIME
  Data Type Conversion6 : DataTypeConversion  OutDataTypeStr=int16  ConvertRealWorld=Stored Integer (SI)  SaturateOnIntegerOverflow=off  RndMeth=Floor
  Demux : Demux  Outputs=2
  Demux1 : Demux  Outputs=2
  FIR Interpolator1 : dsphdlfiltering2/FIR Interpolator  Numerator=TX_INTER.Numerator  FilterStructure=Direct form systolic  InterpolationFactor=TX_INTER.InterpolationFactor  NumCycles=1  SimulateUsing=Code generation  roundingMode=Round  overflowMode=on  CoefficientsDataTypeStr=fixdt(1,16,15)  OutputDataTypeStr=fixdt(1,16,15)  ResetInputPort=off  HDLGlobalReset=off
  Terminator6 : Terminator
  data I out : Outport
  data Q out : Outport  Port=2
  data valid : Outport  Port=3
  wires:
  Complex to Real-Imag/1 -> Demux/1
  Complex to Real-Imag/2 -> Demux1/1
  Data Type Conversion6/1 -> Complex to Real-Imag/1
  FIR Interpolator1/2 -> data valid/1
  FIR Interpolator1/1 -> Data Type Conversion6/1
  Demux/2 -> Bit Concat/1
  Demux/1 -> Bit Concat/2
  Demux1/1 -> Bit Concat1/2
  Demux1/2 -> Bit Concat1/1
  Bit Concat1/1 -> data Q out/1
  Bit Concat/1 -> data I out/1
  FIR Interpolator1/3 -> Terminator6/1
  Constant7/1 -> FIR Interpolator1/2
  data in/1 -> FIR Interpolator1/1

== matlab function QuinReader_HW/MATLAB Function2 ==
  data: SSBnXTsamp input; K1 output; SSdoo input; SSKp input; K2 output
function [K1, K2] = SSPiLoopConstants(SSBnXTsamp, SSdoo, SSKp)
% Compute the constants for the symbol synchronizer loop filter (a PI
% controller)
%
% Inputs:
% SSBnXTsamp -> BnTs/Nsps. BnTs is the noise bandwidth (Bn) normalized to
%   symbol rate (1/Ts). We know that symbol rate 1/Ts equals 2*BLF. Nsps is
%   the number of samples per symbol which equals 4 in our implementation.
%   Noise bandwidth is the most important parameter for us to tune and is
%   not easily acquired. EPC protocol defines the maximum clock drift for
%   each data rate, however it is not enough to help us find the noise
%   bandwidth. Therefore this value is usually acquired through
%   experiments. Anyway, let's say the actual noise bandwidth is alpha*BLF,
%   then we acquire the SSBnXTsamp to be alpha/8. Tuning of this parameter
%   is based on guessing of the alpha.
% SSdoo -> Damping factor, also the zeta in Equation C.57. The PI loop is a
%   second order system and this value is the damping factor for this
%   system. zeta < 1 is underdamped, zeta = 1 is critically damped, and
%   zeta > 1 is overdamped. Typically, it is said that zeta = 1 should
%   generally work. This value might also require tuning, but change this
%   value at last.
% SSKp -> TED Gain. TED produces an error signal once every symbol. It
%   produces a signal that is a function of the timing error tau_e, just
%   like the phase detector in PLL. The characteristic of the TED are
%   described by the S-curve g(tau_e). It means that for if an input signal
%   to TED has a timing error of tar_e, then TED outputs g(tau_e). S-curve
%   is actually computed as the expected value of the error signal for
%   given timing error. When we analyze the S-curve, tau_e is usually
%   normalized to (-0.5, 0.5) using either Ts or Nsps, and the independent
%   variable for g function is the normalized tau_e while the dependent
%   variable is the error signal g. For GTED, S-curve function g is
%   computed as:
%     g = (4 * K^2 * Ex) * C * sin(2 * pi * tau_e / Nsps);
%   where K is the amplitude gain and Ex is the average symbol energy, the
%   channel equalizer equalizes the signal to -1 and 1 PAM, so both should
%   be set to 1. Nsps is still the number of samples per symbol, 4 in our
%   implementation. C is another constant here and is computed as:
%     C = sin(pi * rollOff / 2) / (4 * pi * (1 - (rollOff^2 / 4)));
%   where the rollOff is the roll off factor of the matching filter, and
%   equals 1 since the filter coefficients is [0.25, 0.25, 0.25, 0.25].
%   Therefore, we can directly calculate the S-curve now and it equals:
%     g = 4 / (3 * pi) * sin(2 * pi * (tau_e / Nsps));
%   Note that in our analysis g is a function of (tau_e / Nsps). The TED
%   gain for any type of TED is defined in the same way, the slope of g(0).
%   Therefore, analytically, Kp shoud be 4 / (3 * pi) * 2 * pi = 8 / 3. It
%   is important to note that loop filter should ensure a proper value of
%   Kp is used and leave it as a constant. It's not suggested to tune this
%   parameter.
%   If you want to learn more or make sure the above analysis is accurate,
%   refer to 8.4.1 of "Digital Communication: A Discrete-Time Approach" and
%   the GitHub repo igorauad/symbol_timing_sync, mainly this three
%   functions: `calcTedKp`, `calcSCurve`, and `simSCurve`.
%
%
    SSth = SSBnXTsamp / (SSdoo + 0.25 / SSdoo);  % theta_n in Equation C.57
    SSd  = 1 + 2 * SSdoo * SSth + SSth ^ 2;      % Denominator of Equation C.56
    SSK0 = -1;                                   % Counter (interpolator controller) gain
    % K1 is loop filter's propagation gain
    K1   = 4 * SSdoo * (SSth/SSd) * (1 / (SSKp*SSK0));
    % K2 is loop filter's integral gain
    K2   = 4 *   (SSth^2 / SSd)   * (1 / (SSKp*SSK0));

end
